simulink model "simlinkdatei_angelos_aufgabe_goto"  (Simulink 7.9)
settings: Solver=ode45  StartTime=0.0  StopTime=10.0  RelTol=1e-3
values from neighbouring files (symbols this model uses):
  k = [0.002, 0.2]    [angelos_aufgabe.m]    (also in angelos_doppelt.m = [5000]; my_ode45_abbruch_event_angelos_aufgabe_got.m)
settings Model: Creator=s67750  LastModifiedBy=s67750

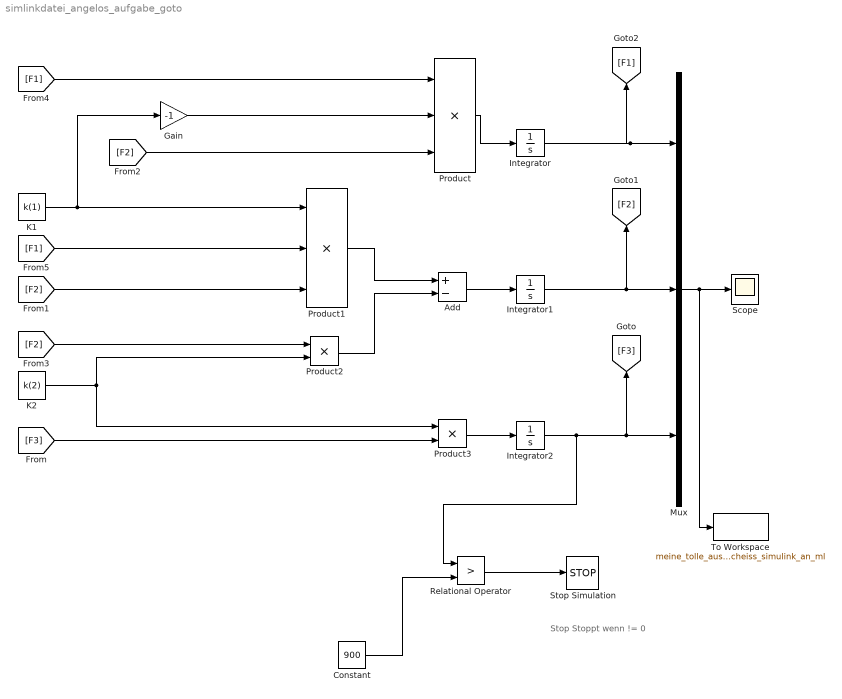
== system simlinkdatei_angelos_aufgabe_goto ==
  note: Stop Stoppt wenn != 0
  Add : Sum  Inputs=+-
  Constant : Constant  Value=900
  Gain : Gain  Gain=-1
  Integrator : Integrator  InitialCondition=1000
  Integrator1 : Integrator  InitialCondition=500
  Integrator2 : Integrator  InitialCondition=200
  K1 : Constant  Value=k(1)
  K2 : Constant  Value=k(2)
  Mux : Mux  Inputs=3
  Product : Product  Inputs=3  RndMeth=Zero
  Product1 : Product  Inputs=3  RndMeth=Zero
  Product2 : Product  RndMeth=Zero
  Product3 : Product  RndMeth=Zero
  Relational Operator : RelationalOperator  Operator=>  OutDataTypeStr=boolean
  Scope : Scope
  Stop Simulation : Stop
  To Workspace : ToWorkspace  VariableName=meine_tolle_ausgabe_von_diesem_scheiss_simulink_an_ml  SampleTime=-1  SaveFormat=Structure With Time
  wires:
  Product2/1 -> Add/2
  Gain/1 -> Product/2
  K1/1 -> Gain/1, Product1/1
  Product/1 -> Integrator/1
  Add/1 -> Integrator1/1
  Product3/1 -> Integrator2/1
  K2/1 -> Product3/1, Product2/2
  Integrator1/1 -> Mux/2, [F2]
  Integrator/1 -> Mux/1, [F1]
  Integrator2/1 -> [F3], Mux/3, Relational Operator/1
  [F3] -> Product3/2
  Mux/1 -> Scope/1, To Workspace/1
  [F2] -> Product1/3
  [F2] -> Product/3
  [F2] -> Product2/1
  [F1] -> Product/1
  Product1/1 -> Add/1
  [F1] -> Product1/2
  Constant/1 -> Relational Operator/2
  Relational Operator/1 -> Stop Simulation/1
